simulink model "mux_demux"  (Simulink 5.0)
settings: Solver=FixedStepDiscrete  StartTime=0.0  StopTime=10.0  RelTol=1e-3
settings Model: Creator=sofronis  LastModifiedBy=sofronis  ExtModeAutoUpdateStatusClock=off  SaveFormat=StructureWithTime  AlgebraicLoopMsg=error

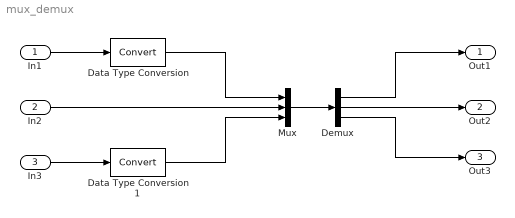
== system mux_demux ==
  In1 : Inport  SampleTime=2
  In2 : Inport  Port=2  SampleTime=2
  In3 : Inport  Port=3  SampleTime=2
  Data Type Conversion : DataTypeConversion  DataType=boolean  SaturateOnIntegerOverflow=on
  Data Type Conversion1 : DataTypeConversion  DataType=uint8  SaturateOnIntegerOverflow=on
  Demux : Demux  Outputs=3
  Mux : Mux  Inputs=3
  Out1 : Outport
  Out2 : Outport  Port=2
  Out3 : Outport  Port=3
  wires:
  In1/1 -> Data Type Conversion/1
  Mux/1 -> Demux/1
  Demux/1 -> Out1/1
  In2/1 -> Mux/2
  In3/1 -> Data Type Conversion1/1
  Demux/2 -> Out2/1
  Demux/3 -> Out3/1
  Data Type Conversion/1 -> Mux/1
  Data Type Conversion1/1 -> Mux/3
